simulink model "Ex20"  (R2019b)
settings: Solver=VariableStepAuto  StartTime=0.0  StopTime=10.0  RelTol=1e-3
values from neighbouring files (symbols this model uses):
  A = 1    [Ex_10.m]    (also in Ex_20.m = 0.1; Ex_28.m = Vf*Wn^2; Ex_29.m = 0.01)
  D = D_v(i)    [Ex_10.m]    (also in Ex_20.m = 3000; Ex_22.m = 0.4; Ex_23.m = 0.1; Ex_29.m = 0.1)
  f = 3    [Ex_20.m]    (also in Ex_21.m; Ex_8.m = [0.1 1 1.6 3 16]*1e3; Ex_9.m = 10.^(1 : 0.01 : 5))
  G = 9.8    [Ex_20.m]    (also in Ex_21.m)
  K1 = 2000    [Ex_20.m]    (also in Ex_24.m = 0.5; Untitled2.m = 1)
  K2 = 25000    [Ex_20.m]    (also in Ex_24.m = 1; Untitled2.m = 1)
  M1 = 400    [Ex_20.m]    (also in Ex_21.m = 0.5; Untitled2.m = 1)
  M2 = 20    [Ex_20.m]    (also in Ex_21.m = 1; Untitled2.m = 1)
settings Model: Creator=andre  LastModifiedBy=andre

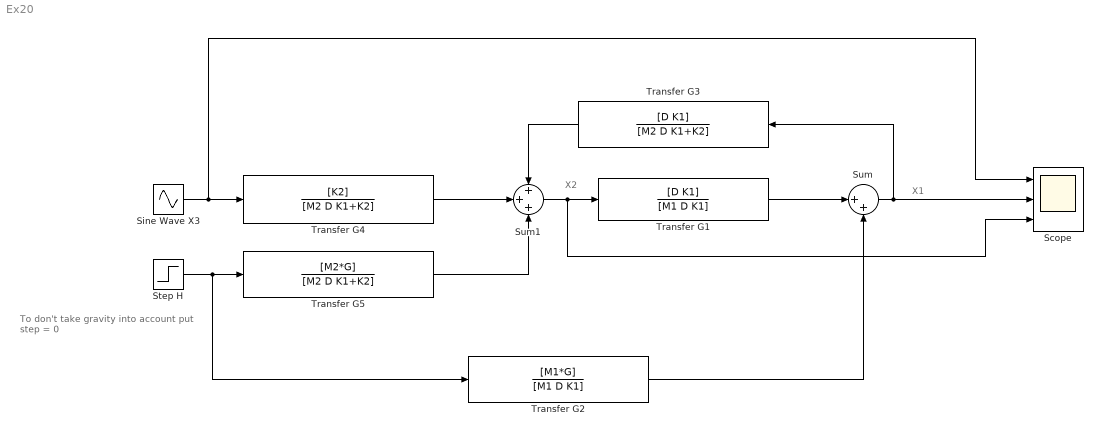
== system Ex20 ==
  note: To don't take gravity into account put step = 0
  note: X1
  note: X2
  Scope : Scope  NumInputPorts=3
  Sine Wave X3 : Sin  Amplitude=A  Frequency=2*pi*f  SampleTime=0
  Step H : Step  Time=0  SampleTime=0
  Sum : Sum  Inputs=|++
  Sum1 : Sum  Inputs=+++
  Transfer G1 : TransferFcn  Numerator=[D K1]  Denominator=[M1 D K1]
  Transfer G2 : TransferFcn  Numerator=[M1*G]  Denominator=[M1 D K1]
  Transfer G3 : TransferFcn  Numerator=[D K1]  Denominator=[M2 D K1+K2]
  Transfer G4 : TransferFcn  Numerator=[K2]  Denominator=[M2 D K1+K2]
  Transfer G5 : TransferFcn  Numerator=[M2*G]  Denominator=[M2 D K1+K2]
  wires:
  Sine Wave X3/1 -> Scope/1, Transfer G4/1
  Step H/1 -> Transfer G2/1, Transfer G5/1
  Sum1/1 -> Scope/3, Transfer G1/1
  Transfer G4/1 -> Sum1/2
  Transfer G5/1 -> Sum1/3
  Transfer G3/1 -> Sum1/1
  Transfer G1/1 -> Sum/1
  Transfer G2/1 -> Sum/2
  Sum/1 -> Transfer G3/1, Scope/2
